simulink model "MS_test"  (R2024b)
settings: Solver=VariableStepAuto  StartTime=0.0  StopTime=10.0  RelTol=1e-3
undefined symbols (not defined in the file): dt, x0
settings Model: Creator=kasek  LastModifiedBy=kseki
settings RTWCC: GPUComputeCapability=3.5

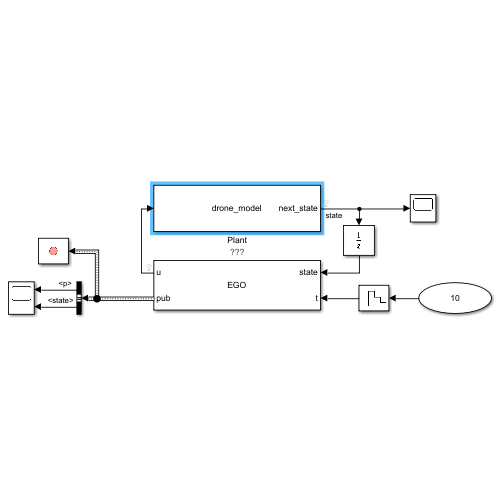
[thumbnail: Simulink's stored preview of the top-level diagram]
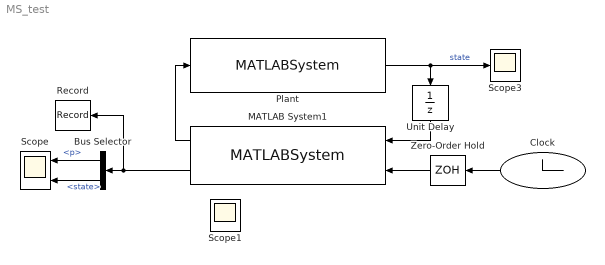
== system MS_test ==
  Bus Selector : BusSelector  OutputSignals=rresult.state.p,eresult.state
  Clock : Clock
  MATLAB System1 : MATLABSystem  System=EGO  SimulateUsing=Code generation
      mask Type: EGO
      mask Display:
      | disp('EGO');
      | port_label('input',1,'state');
      | port_label('input',2,'t');
      | port_label('output',1,'u');
      | port_label('output',2,'pub');
  Plant : MATLABSystem  System=drone_model  SimulateUsing=Code generation
      settings: AttributesFormatString=%<A>
      mask Type: drone_model
      mask Display:
      | disp('drone_model');
      | port_label('output',1,'next_state');
  Record : Record  FileSettingsInternal="{\"entries\":[{\"content\":{\"excelSettings\":{\"content\":{},\"type\":\"Streamout.ExcelSettings\"}},\"type\":\"Streamout.FileSettingStorage\",\"uuid\":\"\"}],\"packageUris\":[\"http:\\/\\/schema.mathworks.com\\/mf0\\/streamout_blocks\\/R2020a\"],\"version\":\"1.0\"}"  SignalsInternal="{\"entries\":[{\"content\":{\"signals\":[{\"content\":{\"blockPath\":[],\"dimensions\":[1,1],\"domain\":\"\",\"hasChildren\":true,\"lineColor\":\"#b746ff\",\"lineWidth\":2,\"port\":1,\"sid\":[\"\"],\"signalID\":1,\"signalName\":\"MATLAB System1:2\"},\"type\":\"RecordBlkView.Signal\",\"uuid\":\"\"},{\"content\":{\"blockPath\":[],\"dimensions\":[1],\"domain\":\"\",\"hasChildren\":true,\"lineColor\":\"#64d413\",\"lineWidth\":2,\"parentID\":1,\"port\":1,\"sid\":[\"\"],\"signalID\":2,\"signalName\":\"rresult\"},\"type\":\"RecordBlkView.Signal\",\"uuid\":\"\"},{\"content\":{\"blockPath\":[],\"dimensions\":[1],\"domain\":\"\",\"hasChildren\":true,\"lineColor\":\"#ff13a6\",\"lineWidth\":2,\"parentID\":2,\"port\":1,\"sid\":[\"\"],\"signalID\":3,\"signalName\":\"state\"},\"type\":\"RecordBlkView.Signal\",\"uuid\":\"\"},{\"content\":{\"blockPath\":[],\"dimensions\":[20,1],\"domain\":\"\",\"hasChildren\":true,\"lineColor\":\"#fe330a\",\"lineWidth\":2,\"parentID\":3,\"port\":1,\"sid\":[\"\"],\"signalID\":4,\"signalName\":\"MATLAB System1:2.rresult.state.xd\"},\"type\":\"RecordBlkView.Signal\",\"uuid\":\"\"},{\"content\":{\"blockPath\":[],\"channel\":[1,1],\"dimensions\":[20,1],\"domain\":\"\",\"leafPath\":\"MATLAB System1:2.rresult.state.xd\",\"lineColor\":\"#77ac30\",\"parentID\":4,\"plots\":[ 1 ],\"port\":1,\"sid\":[\"\"],\"signalID\":5,\"signalName\":\"MATLAB System1:2.rresult.state.xd\"},\"type\":\"RecordBlkView.Signal\",\"uuid\":\"\"},{\"content\":{\"blockPath\":[],\"dimensions\":[3,1],\"domain\":\"\",\"hasChildren\":true,\"lineColor\":\"#0072bd\",\"lineWidth\":2,\"parentID\":3,\"port\":1,\"sid\":[\"\"],\"signalID\":6,\"signalName\":\"MATLAB System1:2.rresult.state.p\"},\"type\":\"RecordBlkView.Signal\",\"uuid\":\"\"},{\"content\":{\"blockPath\":[],\"channel\":[1,1],\"dimensions\":[3,1],\"domain\":\"\",\"leafPath\":\"MATLAB System1:2.rresult.state.p\",\"lineColor\":\"#a2142f\",\"parentID\":6,\"plots\":[ 1 ],\"port\":1,\"sid\":[\"\"],\"signalID\":7,\"signalName\":\"MATLAB System1:2.rresult.state.p\"},\"type\":\"RecordBlkView.Signal\",\"uuid\":\"\"},{\"content\":{\"blockPath\":[],\"dimensions\":[3,1],\"domain\":\"\",\"hasChildren\":true,\"lineColor\":\"#edb120\",\"lineWidth\":2,\"parentID\":3,\"port\":1,\"sid\":[\"\"],\"signalID\":8,\"signalName\":\"MATLAB System1:2.rresult.state.v\"},\"type\":\"RecordBlkView.Signal\",\"uuid\":\"\"},{\"content\":{\"blockPath\":[],\"channel\":[1,1],\"dimensions\":[3,1],\"domain\":\"\",\"leafPath\":\"MATLAB System1:2.rresult.state.v\",\"lineColor\":\"#ff6929\",\"parentID\":8,\"plots\":[ 1 ],\"port\":1,\"sid\":[\"\"],\"signalID\":9,\"signalName\":\"MATLAB System1:2.rresult.state.v\"},\"type\":\"RecordBlkView.Signal\",\"uuid\":\"\"},{\"content\":{\"blockPath\":[],\"dimensions\":[3,1],\"domain\":\"\",\"hasChildren\":true,\"lineColor\":\"#77ac30\",\"lineWidth\":2,\"parentID\":3,\"port\":1,\"sid\":[\"\"],\"signalID\":10,\"signalName\":\"MATLAB System1:2.rresult.state.q\"},\"type\":\"RecordBlkView.Signal\",\"uuid\":\"\"},{\"content\":{\"blockPath\":[],\"channel\":[1,1],\"dimensions\":[3,1],\"domain\":\"\",\"leafPath\":\"MATLAB System1:2.rresult.state.q\",\"lineColor\":\"#64d413\",\"parentID\":10,\"plots\":[ 1 ],\"port\":1,\"sid\":[\"\"],\"signalID\":11,\"signalName\":\"MATLAB System1:2.rresult.state.q\"},\"type\":\"RecordBlkView.Signal\",\"uuid\":\"\"},{\"content\":{\"blockPath\":[],\"dimensions\":[1],\"domain\":\"\",\"hasChildren\":true,\"lineColor\":\"#a2142f\",\"lineWidth\":2,\"parentID\":1,\"port\":1,\"sid\":[\"\"],\"signalID\":12,\"signalName\":\"eresult\"},\"type\":\"RecordBlkView.Signal\",\"uuid\":\"\"},{\"content\":{\"blockPath\":[],\"dimensions\":[12,1],\"domain\":\"\",\"hasChildren\":true,\"lineColor\":\"#139fff\",\"lineWidth\":2,\"parentID\":12,\"port\":1,\"sid\":[\"\"],\"signalID\":13,\"signalName\":\"MATLAB System1:2.eresult.state\"},\"type\":\"RecordBlkView.Signal\",\"uuid\":\"\"},{\"content\":{\"blockPath\":[],\"channel\":[1,1],\"dimensions\":[12,1],\"domain\":\"\",\"leafPath\":\"MATLAB System1:2.eresult.state\",\"lineColor\":\"#22b573\",\"parentID\":13,\"plots\":[ 1 ],\"port\":1,\"sid\":[\"\"],\"signalID\":14,\"signalName\":\"MATLAB System1:2.eresult.state\"},\"type\":\"RecordBlkView.Signal\",\"uuid\":\"\"},{\"content\":{\"blockPath\":[],\"dimensions\":[12,12],\"domain\":\"\",\"hasChildren\":true,\"lineColor\":\"#b746ff\",\"lineWidth\":2,\"parentID\":12,\"port\":1,\"sid\":[\"\"],\"signalID\":15,\"signalName\":\"MATLAB System1:2.eresult.P\"},\"type\":\"RecordBlkView.Signal\",\"uuid\":\"\"},{\"content\":{\"blockPath\":[],\"channel\":[1,1],\"dimensions\":[12,12],\"domain\":\"\",\"leafPath\":\"MATLAB System1:2.eresult.P\",\"lineColor\":\"#d95319\",\"parentID\":15,\"plots\":[ 1 ],\"port\":1,\"sid\":[\"\"],\"signalID\":16,\"signalName\":\"MATLAB System1:2.eresult.P\"},\"type\":\"RecordBlkView.Signal\",\"uuid\":\"\"},{\"content\":{\"blockPath\":[],\"dimensions\":[1],\"domain\":\"\",\"hasChildren\":true,\"lineColor\":\"#ff13a6\",\"lineWidth\":2,\"parentID\":1,\"port\":1,\"sid\":[\"\"],\"signalID\":17,\"signalName\":\"cresult\"},\"type\":\"RecordBlkView.Signal\",\"uuid\":\"\"},{\"content\":{\"blockPath\":[],\"dimensions\":[4,1],\"domain\":\"\",\"hasChildren\":true,\"lineColor\":\"#fe330a\",\"lineWidth\":2,\"parentID\":17,\"port\":1,\"sid\":[\"\"],\"signalID\":18,\"signalName\":\"MATLAB System1:2.cresult.input\"},\"type\":\"RecordBlkView.Signal\",\"uuid\":\"\"},{\"content\":{\"blockPath\":[],\"channel\":[1,1],\"dimensions\":[4,1],\"domain\":\"\",\"leafPath\":\"MATLAB System1:2.cresult.input\",\"lineColor\":\"#77ac30\",\"parentID\":18,\"plots\":[ 1 ],\"port\":1,\"sid\":[\"\"],\"signalID\":19,\"signalName\":\"MATLAB System1:2.cresult.input\"},\"type\":\"RecordBlkView.Signal\",\"uuid\":\"\"},{\"content\":{\"blockPath\":[],\"channel\":[2,1],\"dimensions\":[3,1],\"domain\":\"\",\"leafPath\":\"MATLAB System1:2.rresult.state.p\",\"lineColor\":\"#ff6929\",\"parentID\":6,\"plots\":[ 1 ],\"port\":1,\"sid\":[\"\"],\"signalID\":20,\"signalName\":\"MATLAB System1:2.rresult.state.p\"},\"type\":\"RecordBlkView.Signal\",\"uuid\":\"\"},{\"content\":{\"blockPath\":[],\"channel\":[3,1],\"dimensions\":[3,1],\"domain\":\"\",\"leafPath\":\"MATLAB System1:2.rresult.state.p\",\"lineColor\":\"#b746ff\",\"parentID\":6,\"plots\":[ 1 ],\"port\":1,\"sid\":[\"\"],\"signalID\":21,\"signalName\":\"MATLAB System1:2.rresult.state.p\"},\"type\":\"RecordBlkView.Signal\",\"uuid\":\"\"},{\"content\":{\"blockPath\":[],\"channel\":[2,1],\"dimensions\":[3,1],\"domain\":\"\",\"leafPath\":\"MATLAB System1:2.rresult.state.v\",\"lineColor\":\"#64d413\",\"parentID\":8,\"plots\":[ 1 ],\"port\":1,\"sid\":[\"\"],\"signalID\":22,\"signalName\":\"MATLAB System1:2.rresult.state.v\"},\"type\":\"RecordBlkView.Signal\",\"uuid\":\"\"},{\"content\":{\"blockPath\":[],\"channel\":[3,1],\"dimensions\":[3,1],\"domain\":\"\",\"leafPath\":\"MATLAB System1:2.rresult.state.v\",\"lineColor\":\"#ff13a6\",\"parentID\":8,\"plots\":[ 1 ],\"port\":1,\"sid\":[\"\"],\"signalID\":23,\"signalName\":\"MATLAB System1:2.rresult.state.v\"},\"type\":\"RecordBlkView.Signal\",\"uuid\":\"\"},{\"content\":{\"blockPath\":[],\"channel\":[2,1],\"dimensions\":[3,1],\"domain\":\"\",\"leafPath\":\"MATLAB System1:2.rresult.state.q\",\"lineColor\":\"#fe330a\",\"parentID\":10,\"plots\":[ 1 ],\"port\":1,\"sid\":[\"\"],\"signalID\":24,\"signalName\":\"MATLAB System1:2.rresult.state.q\"},\"type\":\"RecordBlkView.Signal\",\"uuid\":\"\"},{\"content\":{\"blockPath\":[],\"channel\":[3,1],\"dimensions\":[3,1],\"domain\":\"\",\"leafPath\":\"MATLAB System1:2.rresult.state.q\",\"lineColor\":\"#22b573\",\"parentID\":10,\"plots\":[ 1 ],\"port\":1,\"sid\":[\"\"],\"signalID\":25,\"signalName\":\"MATLAB System1:2.rresult.state.q\"},\"type\":\"RecordBlkView.Signal\",\"uuid\":\"\"},{\"content\":{\"blockPath\":[],\"channel\":[2,1],\"dimensions\":[4,1],\"domain\":\"\",\"leafPath\":\"MATLAB System1:2.cresult.input\",\"lineColor\":\"#0072bd\",\"parentID\":18,\"plots\":[ 1 ],\"port\":1,\"sid\":[\"\"],\"signalID\":26,\"signalName\":\"MATLAB System1:2.cresult.input\"},\"type\":\"RecordBlkView.Signal\",\"uuid\":\"\"},{\"content\":{\"blockPath\":[],\"channel\":[3,1],\"dimensions\":[4,1],\"domain\":\"\",\"leafPath\":\"MATLAB System1:2.cresult.input\",\"lineColor\":\"#d95319\",\"parentID\":18,\"plots\":[ 1 ],\"port\":1,\"sid\":[\"\"],\"signalID\":27,\"signalName\":\"MATLAB System1:2.cresult.input\"},\"type\":\"RecordBlkView.Signal\",\"uuid\":\"\"},{\"content\":{\"blockPath\":[],\"channel\":[4,1],\"dimensions\":[4,1],\"domain\":\"\",\"leafPath\":\"MATLAB System1:2.cresult.input\",\"lineColor\":\"#edb120\",\"parentID\":18,\"plots\":[ 1 ],\"port\":1,\"sid\":[\"\"],\"signalID\":28,\"signalName\":\"MATLAB System1:2.cresult.input\"},\"type\":\"RecordBlkView.Signal\",\"uuid\":\"\"},{\"content\":{\"blockPath\":[],\"channel\":[2,1],\"dimensions\":[20,1],\"domain\":\"\",\"leafPath\":\"MATLAB System1:2.rresult.state.xd\",\"lineColor\":\"#fe330a\",\"lineWidth\":2,\"parentID\":4,\"plots\":[ 1 ],\"port\":1,\"sid\":[\"\"],\"signalID\":29,\"signalName\":\"MATLAB System1:2.rresult.state.xd\"},\"type\":\"RecordBlkView.Signal\",\"uuid\":\"\"},{\"content\":{\"blockPath\":[],\"channel\":[3,1],\"dimensions\":[20,1],\"domain\":\"\",\"leafPath\":\"MATLAB System1:2.rresult.state.xd\",\"lineColor\":\"#22b573\",\"lineWidth\":2,\"parentID\":4,\"plots\":[ 1 ],\"port\":1,\"sid\":[\"\"],\"signalID\":30,\"signalName\":\"MATLAB System1:2.rresult.state.xd\"},\"type\":\"RecordBlkView.Signal\",\"uuid\":\"\"},{\"content\":{\"blockPath\":[],\"channel\":[4,1],\"dimensions\":[20,1],\"domain\":\"\",\"leafPath\":\"MATLAB System1:2.rresult.state.xd\",\"lineColor\":\"#0072bd\",\"lineWidth\":2,\"parentID\":4,\"plots\":[ 1 ],\"port\":1,\"sid\":[\"\"],\"signalID\":31,\"signalName\":\"MATLAB System1:2.rresult.state.xd\"},\"type\":\"RecordBlkView.Signal\",\"uuid\":\"\"},{\"content\":{\"blockPath\":[],\"channel\":[5,1],\"dimensions\":[20,1],\"domain\":\"\",\"leafPath\":\"MATLAB System1:2.rresult.state.xd\",\"lineColor\":\"#d95319\",\"lineWidth\":2,\"parentID\":4,\"port\":1,\"sid\":[\"\"],\"signalID\":32,\"signalName\":\"MATLAB System1:2.rresult.state.xd\"},\"type\":\"RecordBlkView.Signal\",\"uuid\":\"\"},{\"content\":{\"blockPath\":[],\"channel\":[6,1],\"dimensions\":[20,1],\"domain\":\"\",\"leafPath\":\"MATLAB System1:2.rresult.state.xd\",\"lineColor\":\"#edb120\",\"lineWidth\":2,\"parentID\":4,\"port\":1,\"sid\":[\"\"],\"signalID\":33,\"signalName\":\"MATLAB System1:2.rresult.state.xd\"},\"type\":\"RecordBlkView.Signal\",\"uuid\":\"\"},{\"content\":{\"blockPath\":[],\"channel\":[7,1],\"dimensions\":[20,1],\"domain\":\"\",\"leafPath\":\"MATLAB System1:2.rresult.state.xd\",\"lineColor\":\"#7e2f8e\",\"lineWidth\":2,\"parentID\":4,\"port\":1,\"sid\":[\"\"],\"signalID\":34,\"signalName\":\"MATLAB System1:2.rresult.state.xd\"},\"type\":\"RecordBlkView.Signal\",\"uuid\":\"\"},{\"content\":{\"blockPath\":[],\"channel\":[8,1],\"dimensions\":[20,1],\"domain\":\"\",\"leafPath\":\"MATLAB System1:2.rresult.state.xd\",\"lineColor\":\"#77ac30\",\"lineWidth\":2,\"parentID\":4,\"port\":1,\"sid\":[\"\"],\"signalID\":35,\"signalName\":\"MATLAB System1:2.rresult.state.xd\"},\"type\":\"RecordBlkView.Signal\",\"uuid\":\"\"},{\"content\":{\"blockPath\":[],\"channel\":[9,1],\"dimensions\":[20,1],\"domain\":\"\",\"leafPath\":\"MATLAB System1:2.rresult.state.xd\",\"lineColor\":\"#4dbeee\",\"lineWidth\":2,\"parentID\":4,\"port\":1,\"sid\":[\"\"],\"signalID\":36,\"signalName\":\"MATLAB System1:2.rresult.state.xd\"},\"type\":\"RecordBlkView.Signal\",\"uuid\":\"\"},{\"content\":{\"blockPath\":[],\"channel\":[10,1],\"dimensions\":[20,1],\"domain\":\"\",\"leafPath\":\"MATLAB System1:2.rresult.state.xd\",\"lineColor\":\"#a2142f\",\"lineWidth\":2,\"parentID\":4,\"port\":1,\"sid\":[\"\"],\"signalID\":37,\"signalName\":\"MATLAB System1:2.rresult.state.xd\"},\"type\":\"RecordBlkView.Signal\",\"uuid\":\"\"},{\"content\":{\"blockPath\":[],\"channel\":[11,1],\"dimensions\":[20,1],\"domain\":\"\",\"leafPath\":\"MATLAB System1:2.rresult.state.xd\",\"lineColor\":\"#139fff\",\"lineWidth\":2,\"parentID\":4,\"port\":1,\"sid\":[\"\"],\"signalID\":38,\"signalName\":\"MATLAB System1:2.rresult.state.xd\"},\"type\":\"RecordBlkView.Signal\",\"uuid\":\"\"},{\"content\":{\"blockPath\":[],\"channel\":[12,1],\"dimensions\":[20,1],\"domain\":\"\",\"leafPath\":\"MATLAB System1:2.rresult.state.xd\",\"lineColor\":\"#ff6929\",\"lineWidth\":2,\"parentID\":4,\"port\":1,\"sid\":[\"\"],\"signalID\":39,\"signalName\":\"MATLAB System1:2.rresult.state.xd\"},\"type\":\"RecordBlkView.Signal\",\"uuid\":\"\"},{\"content\":{\"blockPath\":[],\"channel\":[13,1],\"dimensions\":[20,1],\"domain\":\"\",\"leafPath\":\"MATLAB System1:2.rresult.state.xd\",\"lineColor\":\"#b746ff\",\"lineWidth\":2,\"parentID\":4,\"port\":1,\"sid\":[\"\"],\"signalID\":40,\"signalName\":\"MATLAB System1:2.rresult.state.xd\"},\"type\":\"RecordBlkView.Signal\",\"uuid\":\"\"},{\"content\":{\"blockPath\":[],\"channel\":[14,1],\"dimensions\":[20,1],\"domain\":\"\",\"leafPath\":\"MATLAB System1:2.rresult.state.xd\",\"lineColor\":\"#64d413\",\"lineWidth\":2,\"parentID\":4,\"port\":1,\"sid\":[\"\"],\"signalID\":41,\"signalName\":\"MATLAB System1:2.rresult.state.xd\"},\"type\":\"RecordBlkView.Signal\",\"uuid\":\"\"},{\"content\":{\"blockPath\":[],\"channel\":[15,1],\"dimensions\":[20,1],\"domain\":\"\",\"leafPath\":\"MATLAB System1:2.rresult.state.xd\",\"lineColor\":\"#ff13a6\",\"lineWidth\":2,\"parentID\":4,\"port\":1,\"sid\":[\"\"],\"signalID\":42,\"signalName\":\"MATLAB System1:2.rresult.state.xd\"},\"type\":\"RecordBlkView.Signal\",\"uuid\":\"\"},{\"content\":{\"blockPath\":[],\"channel\":[16,1],\"dimensions\":[20,1],\"domain\":\"\",\"leafPath\":\"MATLAB System1:2.rresult.state.xd\",\"lineColor\":\"#fe330a\",\"lineWidth\":2,\"parentID\":4,\"port\":1,\"sid\":[\"\"],\"signalID\":43,\"signalName\":\"MATLAB System1:2.rresult.state.xd\"},\"type\":\"RecordBlkView.Signal\",\"uuid\":\"\"},{\"content\":{\"blockPath\":[],\"channel\":[17,1],\"dimensions\":[20,1],\"domain\":\"\",\"leafPath\":\"MATLAB System1:2.rresult.state.xd\",\"lineColor\":\"#22b573\",\"lineWidth\":2,\"parentID\":4,\"port\":1,\"sid\":[\"\"],\"signalID\":44,\"signalName\":\"MATLAB System1:2.rresult.state.xd\"},\"type\":\"RecordBlkView.Signal\",\"uuid\":\"\"},{\"content\":{\"blockPath\":[],\"channel\":[18,1],\"dimensions\":[20,1],\"domain\":\"\",\"leafPath\":\"MATLAB System1:2.rresult.state.xd\",\"lineColor\":\"#0072bd\",\"lineWidth\":2,\"parentID\":4,\"port\":1,\"sid\":[\"\"],\"signalID\":45,\"signalName\":\"MATLAB System1:2.rresult.state.xd\"},\"type\":\"RecordBlkView.Signal\",\"uuid\":\"\"},{\"content\":{\"blockPath\":[],\"channel\":[19,1],\"dimensions\":[20,1],\"domain\":\"\",\"leafPath\":\"MATLAB System1:2.rresult.state.xd\",\"lineColor\":\"#d95319\",\"lineWidth\":2,\"parentID\":4,\"port\":1,\"sid\":[\"\"],\"signalID\":46,\"signalName\":\"MATLAB System1:2.rresult.state.xd\"},\"type\":\"RecordBlkView.Signal\",\"uuid\":\"\"},{\"content\":{\"blockPath\":[],\"channel\":[20,1],\"dimensions\":[20,1],\"domain\":\"\",\"leafPath\":\"MATLAB System1:2.rresult.state.xd\",\"lineColor\":\"#edb120\",\"lineWidth\":2,\"parentID\":4,\"port\":1,\"sid\":[\"\"],\"signalID\":47,\"signalName\":\"MATLAB System1:2.rresult.state.xd\"},\"type\":\"RecordBlkView.Signal\",\"uuid\":\"\"},{\"content\":{\"blockPath\":[],\"channel\":[2,1],\"dimensions\":[12,1],\"domain\":\"\",\"leafPath\":\"MATLAB System1:2.eresult.state\",\"lineColor\":\"#7e2f8e\",\"lineWidth\":2,\"parentID\":13,\"plots\":[ 1 ],\"port\":1,\"sid\":[\"\"],\"signalID\":48,\"signalName\":\"MATLAB System1:2.eresult.state\"},\"type\":\"RecordBlkView.Signal\",\"uuid\":\"\"},{\"content\":{\"blockPath\":[],\"channel\":[3,1],\"dimensions\":[12,1],\"domain\":\"\",\"leafPath\":\"MATLAB System1:2.eresult.state\",\"lineColor\":\"#77ac30\",\"lineWidth\":2,\"parentID\":13,\"plots\":[ 1 ],\"port\":1,\"sid\":[\"\"],\"signalID\":49,\"signalName\":\"MATLAB System1:2.eresult.state\"},\"type\":\"RecordBlkView.Signal\",\"uuid\":\"\"},{\"content\":{\"blockPath\":[],\"channel\":[4,1],\"dimensions\":[12,1],\"domain\":\"\",\"leafPath\":\"MATLAB System1:2.eresult.state\",\"lineColor\":\"#4dbeee\",\"lineWidth\":2,\"parentID\":13,\"plots\":[ 1 ],\"port\":1,\"sid\":[\"\"],\"signalID\":50,\"signalName\":\"MATLAB System1:2.eresult.state\"},\"type\":\"RecordBlkView.Signal\",\"uuid\":\"\"},{\"content\":{\"blockPath\":[],\"channel\":[5,1],\"dimensions\":[12,1],\"domain\":\"\",\"leafPath\":\"MATLAB System1:2.eresult.state\",\"lineColor\":\"#a2142f\",\"lineWidth\":2,\"parentID\":13,\"port\":1,\"sid\":[\"\"],\"signalID\":51,\"signalName\":\"MATLAB System1:2.eresult.state\"},\"type\":\"RecordBlkView.Signal\",\"uuid\":\"\"},{\"content\":{\"blockPath\":[],\"channel\":[6,1],\"dimensions\":[12,1],\"domain\":\"\",\"leafPath\":\"MATLAB System1:2.eresult.state\",\"lineColor\":\"#139fff\",\"lineWidth\":2,\"parentID\":13,\"port\":1,\"sid\":[\"\"],\"signalID\":52,\"signalName\":\"MATLAB System1:2.eresult.state\"},\"type\":\"RecordBlkView.Signal\",\"uuid\":\"\"},{\"content\":{\"blockPath\":[],\"channel\":[7,1],\"dimensions\":[12,1],\"domain\":\"\",\"leafPath\":\"MATLAB System1:2.eresult.state\",\"lineColor\":\"#ff6929\",\"lineWidth\":2,\"parentID\":13,\"port\":1,\"sid\":[\"\"],\"signalID\":53,\"signalName\":\"MATLAB System1:2.eresult.state\"},\"type\":\"RecordBlkView.Signal\",\"uuid\":\"\"},{\"content\":{\"blockPath\":[],\"channel\":[8,1],\"dimensions\":[12,1],\"domain\":\"\",\"leafPath\":\"MATLAB System1:2.eresult.state\",\"lineColor\":\"#b746ff\",\"lineWidth\":2,\"parentID\":13,\"port\":1,\"sid\":[\"\"],\"signalID\":54,\"signalName\":\"MATLAB System1:2.eresult.state\"},\"type\":\"RecordBlkView.Signal\",\"uuid\":\"\"},{\"content\":{\"blockPath\":[],\"channel\":[9,1],\"dimensions\":[12,1],\"domain\":\"\",\"leafPath\":\"MATLAB System1:2.eresult.state\",\"lineColor\":\"#64d413\",\"lineWidth\":2,\"parentID\":13,\"port\":1,\"sid\":[\"\"],\"signalID\":55,\"signalName\":\"MATLAB System1:2.eresult.state\"},\"type\":\"RecordBlkView.Signal\",\"uuid\":\"\"},{\"content\":{\"blockPath\":[],\"channel\":[10,1],\"dimensions\":[12,1],\"domain\":\"\",\"leafPath\":\"MATLAB System1:2.eresult.state\",\"lineColor\":\"#ff13a6\",\"lineWidth\":2,\"parentID\":13,\"port\":1,\"sid\":[\"\"],\"signalID\":56,\"signalName\":\"MATLAB System1:2.eresult.state\"},\"type\":\"RecordBlkView.Signal\",\"uuid\":\"\"},{\"content\":{\"blockPath\":[],\"channel\":[11,1],\"dimensions\":[12,1],\"domain\":\"\",\"leafPath\":\"MATLAB System1:2.eresult.state\",\"lineColor\":\"#fe330a\",\"lineWidth\":2,\"parentID\":13,\"port\":1,\"sid\":[\"\"],\"signalID\":57,\"signalName\":\"MATLAB System1:2.eresult.state\"},\"type\":\"RecordBlkView.Signal\",\"uuid\":\"\"},{\"content\":{\"blockPath\":[],\"channel\":[12,1],\"dimensions\":[12,1],\"domain\":\"\",\"leafPath\":\"MATLAB System1:2.eresult.state\",\"lineColor\":\"#22b573\",\"lineWidth\":2,\"parentID\":13,\"port\":1,\"sid\":[\"\"],\"signalID\":58,\"signalName\":\"MATLAB System1:2.eresult.state\"},\"type\":\"RecordBlkView.Signal\",\"uuid\":\"\"},{\"content\":{\"blockPath\":[],\"channel\":[2,1],\"dimensions\":[12,12],\"domain\":\"\",\"leafPath\":\"MATLAB System1:2.eresult.P\",\"lineColor\":\"#0072bd\",\"lineWidth\":2,\"parentID\":15,\"plots\":[ 1 ],\"port\":1,\"sid\":[\"\"],\"signalID\":59,\"signalName\":\"MATLAB System1:2.eresult.P\"},\"type\":\"RecordBlkView.Signal\",\"uuid\":\"\"},{\"content\":{\"blockPath\":[],\"channel\":[3,1],\"dimensions\":[12,12],\"domain\":\"\",\"leafPath\":\"MATLAB System1:2.eresult.P\",\"lineColor\":\"#d95319\",\"lineWidth\":2,\"parentID\":15,\"plots\":[ 1 ],\"port\":1,\"sid\":[\"\"],\"signalID\":60,\"signalName\":\"MATLAB System1:2.eresult.P\"},\"type\":\"RecordBlkView.Signal\",\"uuid\":\"\"},{\"content\":{\"blockPath\":[],\"channel\":[4,1],\"dimensions\":[12,12],\"domain\":\"\",\"leafPath\":\"MATLAB System1:2.eresult.P\",\"lineColor\":\"#edb120\",\"lineWidth\":2,\"parentID\":15,\"plots\":[ 1 ],\"port\":1,\"sid\":[\"\"],\"signalID\":61,\"signalName\":\"MATLAB System1:2.eresult.P\"},\"type\":\"RecordBlkView.Signal\",\"uuid\":\"\"},{\"content\":{\"blockPath\":[],\"channel\":[5,1],\"dimensions\":[12,12],\"domain\":\"\",\"leafPath\":\"MATLAB System1:2.eresult.P\",\"lineColor\":\"#7e2f8e\",\"lineWidth\":2,\"parentID\":15,\"port\":1,\"sid\":[\"\"],\"signalID\":62,\"signalName\":\"MATLAB System1:2.eresult.P\"},\"type\":\"RecordBlkView.Signal\",\"uuid\":\"\"},{\"content\":{\"blockPath\":[],\"channel\":[6,1],\"dimensions\":[12,12],\"domain\":\"\",\"leafPath\":\"MATLAB System1:2.eresult.P\",\"lineColor\":\"#77ac30\",\"lineWidth\":2,\"parentID\":15,\"port\":1,\"sid\":[\"\"],\"signalID\":63,\"signalName\":\"MATLAB System1:2.eresult.P\"},\"type\":\"RecordBlkView.Signal\",\"uuid\":\"\"},{\"content\":{\"blockPath\":[],\"channel\":[7,1],\"dimensions\":[12,12],\"domain\":\"\",\"leafPath\":\"MATLAB System1:2.eresult.P\",\"lineColor\":\"#4dbeee\",\"lineWidth\":2,\"parentID\":15,\"port\":1,\"sid\":[\"\"],\"signalID\":64,\"signalName\":\"MATLAB System1:2.eresult.P\"},\"type\":\"RecordBlkView.Signal\",\"uuid\":\"\"},{\"content\":{\"blockPath\":[],\"channel\":[8,1],\"dimensions\":[12,12],\"domain\":\"\",\"leafPath\":\"MATLAB System1:2.eresult.P\",\"lineColor\":\"#a2142f\",\"lineWidth\":2,\"parentID\":15,\"port\":1,\"sid\":[\"\"],\"signalID\":65,\"signalName\":\"MATLAB System1:2.eresult.P\"},\"type\":\"RecordBlkView.Signal\",\"uuid\":\"\"},{\"content\":{\"blockPath\":[],\"channel\":[9,1],\"dimensions\":[12,12],\"domain\":\"\",\"leafPath\":\"MATLAB System1:2.eresult.P\",\"lineColor\":\"#139fff\",\"lineWidth\":2,\"parentID\":15,\"port\":1,\"sid\":[\"\"],\"signalID\":66,\"signalName\":\"MATLAB System1:2.eresult.P\"},\"type\":\"RecordBlkView.Signal\",\"uuid\":\"\"},{\"content\":{\"blockPath\":[],\"channel\":[10,1],\"dimensions\":[12,12],\"domain\":\"\",\"leafPath\":\"MATLAB System1:2.eresult.P\",\"lineColor\":\"#ff6929\",\"lineWidth\":2,\"parentID\":15,\"port\":1,\"sid\":[\"\"],\"signalID\":67,\"signalName\":\"MATLAB System1:2.eresult.P\"},\"type\":\"RecordBlkView.Signal\",\"uuid\":\"\"},{\"content\":{\"blockPath\":[],\"channel\":[11,1],\"dimensions\":[12,12],\"domain\":\"\",\"leafPath\":\"MATLAB System1:2.eresult.P\",\"lineColor\":\"#b746ff\",\"lineWidth\":2,\"parentID\":15,\"port\":1,\"sid\":[\"\"],\"signalID\":68,\"signalName\":\"MATLAB System1:2.eresult.P\"},\"type\":\"RecordBlkView.Signal\",\"uuid\":\"\"},{\"content\":{\"blockPath\":[],\"channel\":[12,1],\"dimensions\":[12,12],\"domain\":\"\",\"leafPath\":\"MATLAB System1:2.eresult.P\",\"lineColor\":\"#64d413\",\"lineWidth\":2,\"parentID\":15,\"port\":1,\"sid\":[\"\"],\"signalID\":69,\"signalName\":\"MATLAB System1:2.eresult.P\"},\"type\":\"RecordBlkView.Signal\",\"uuid\":\"\"},{\"content\":{\"blockPath\":[],\"channel\":[1,2],\"dimensions\":[12,12],\"domain\":\"\",\"leafPath\":\"MATLAB System1:2.eresult.P\",\"lineColor\":\"#ff13a6\",\"lineWidth\":2,\"parentID\":15,\"port\":1,\"sid\":[\"\"],\"signalID\":70,\"signalName\":\"MATLAB System1:2.eresult.P\"},\"type\":\"RecordBlkView.Signal\",\"uuid\":\"\"},{\"content\":{\"blockPath\":[],\"channel\":[2,2],\"dimensions\":[12,12],\"domain\":\"\",\"leafPath\":\"MATLAB System1:2.eresult.P\",\"lineColor\":\"#fe330a\",\"lineWidth\":2,\"parentID\":15,\"port\":1,\"sid\":[\"\"],\"signalID\":71,\"signalName\":\"MATLAB System1:2.eresult.P\"},\"type\":\"RecordBlkView.Signal\",\"uuid\":\"\"},{\"content\":{\"blockPath\":[],\"channel\":[3,2],\"dimensions\":[12,12],\"domain\":\"\",\"leafPath\":\"MATLAB System1:2.eresult.P\",\"lineColor\":\"#22b573\",\"lineWidth\":2,\"parentID\":15,\"port\":1,\"sid\":[\"\"],\"signalID\":72,\"signalName\":\"MATLAB System1:2.eresult.P\"},\"type\":\"RecordBlkView.Signal\",\"uuid\":\"\"},{\"content\":{\"blockPath\":[],\"channel\":[4,2],\"dimensions\":[12,12],\"domain\":\"\",\"leafPath\":\"MATLAB System1:2.eresult.P\",\"lineColor\":\"#0072bd\",\"lineWidth\":2,\"parentID\":15,\"port\":1,\"sid\":[\"\"],\"signalID\":73,\"signalName\":\"MATLAB System1:2.eresult.P\"},\"type\":\"RecordBlkView.Signal\",\"uuid\":\"\"},{\"content\":{\"blockPath\":[],\"channel\":[5,2],\"dimensions\":[12,12],\"domain\":\"\",\"leafPath\":\"MATLAB System1:2.eresult.P\",\"lineColor\":\"#d95319\",\"lineWidth\":2,\"parentID\":15,\"port\":1,\"sid\":[\"\"],\"signalID\":74,\"signalName\":\"MATLAB System1:2.eresult.P\"},\"type\":\"RecordBlkView.Signal\",\"uuid\":\"\"},{\"content\":{\"blockPath\":[],\"channel\":[6,2],\"dimensions\":[12,12],\"domain\":\"\",\"leafPath\":\"MATLAB System1:2.eresult.P\",\"lineColor\":\"#edb120\",\"lineWidth\":2,\"parentID\":15,\"port\":1,\"sid\":[\"\"],\"signalID\":75,\"signalName\":\"MATLAB System1:2.eresult.P\"},\"type\":\"RecordBlkView.Signal\",\"uuid\":\"\"},{\"content\":{\"blockPath\":[],\"channel\":[7,2],\"dimensions\":[12,12],\"domain\":\"\",\"leafPath\":\"MATLAB System1:2.eresult.P\",\"lineColor\":\"#7e2f8e\",\"lineWidth\":2,\"parentID\":15,\"port\":1,\"sid\":[\"\"],\"signalID\":76,\"signalName\":\"MATLAB System1:2.eresult.P\"},\"type\":\"RecordBlkView.Signal\",\"uuid\":\"\"},{\"content\":{\"blockPath\":[],\"channel\":[8,2],\"dimensions\":[12,12],\"domain\":\"\",\"leafPath\":\"MATLAB System1:2.eresult.P\",\"lineColor\":\"#77ac30\",\"lineWidth\":2,\"parentID\":15,\"port\":1,\"sid\":[\"\"],\"signalID\":77,\"signalName\":\"MATLAB System1:2.eresult.P\"},\"type\":\"RecordBlkView.Signal\",\"uuid\":\"\"},{\"content\":{\"blockPath\":[],\"channel\":[9,2],\"dimensions\":[12,12],\"domain\":\"\",\"leafPath\":\"MATLAB System1:2.eresult.P\",\"lineColor\":\"#4dbeee\",\"lineWidth\":2,\"parentID\":15,\"port\":1,\"sid\":[\"\"],\"signalID\":78,\"signalName\":\"MATLAB System1:2.eresult.P\"},\"type\":\"RecordBlkView.Signal\",\"uuid\":\"\"},{\"content\":{\"blockPath\":[],\"channel\":[10,2],\"dimensions\":[12,12],\"domain\":\"\",\"leafPath\":\"MATLAB System1:2.eresult.P\",\"lineColor\":\"#a2142f\",\"lineWidth\":2,\"parentID\":15,\"port\":1,\"sid\":[\"\"],\"signalID\":79,\"signalName\":\"MATLAB System1:2.eresult.P\"},\"type\":\"RecordBlkView.Signal\",\"uuid\":\"\"},{\"content\":{\"blockPath\":[],\"channel\":[11,2],\"dimensions\":[12,12],\"domain\":\"\",\"leafPath\":\"MATLAB System1:2.eresult.P\",\"lineColor\":\"#139fff\",\"lineWidth\":2,\"parentID\":15,\"port\":1,\"sid\":[\"\"],\"signalID\":80,\"signalName\":\"MATLAB System1:2.eresult.P\"},\"type\":\"RecordBlkView.Signal\",\"uuid\":\"\"},{\"content\":{\"blockPath\":[],\"channel\":[12,2],\"dimensions\":[12,12],\"domain\":\"\",\"leafPath\":\"MATLAB System1:2.eresult.P\",\"lineColor\":\"#ff6929\",\"lineWidth\":2,\"parentID\":15,\"port\":1,\"sid\":[\"\"],\"signalID\":81,\"signalName\":\"MATLAB System1:2.eresult.P\"},\"type\":\"RecordBlkView.Signal\",\"uuid\":\"\"},{\"content\":{\"blockPath\":[],\"channel\":[1,3],\"dimensions\":[12,12],\"domain\":\"\",\"leafPath\":\"MATLAB System1:2.eresult.P\",\"lineColor\":\"#b746ff\",\"lineWidth\":2,\"parentID\":15,\"port\":1,\"sid\":[\"\"],\"signalID\":82,\"signalName\":\"MATLAB System1:2.eresult.P\"},\"type\":\"RecordBlkView.Signal\",\"uuid\":\"\"},{\"content\":{\"blockPath\":[],\"channel\":[2,3],\"dimensions\":[12,12],\"domain\":\"\",\"leafPath\":\"MATLAB System1:2.eresult.P\",\"lineColor\":\"#64d413\",\"lineWidth\":2,\"parentID\":15,\"port\":1,\"sid\":[\"\"],\"signalID\":83,\"signalName\":\"MATLAB System1:2.eresult.P\"},\"type\":\"RecordBlkView.Signal\",\"uuid\":\"\"},{\"content\":{\"blockPath\":[],\"channel\":[3,3],\"dimensions\":[12,12],\"domain\":\"\",\"leafPath\":\"MATLAB System1:2.eresult.P\",\"lineColor\":\"#ff13a6\",\"lineWidth\":2,\"parentID\":15,\"port\":1,\"sid\":[\"\"],\"signalID\":84,\"signalName\":\"MATLAB System1:2.eresult.P\"},\"type\":\"RecordBlkView.Signal\",\"uuid\":\"\"},{\"content\":{\"blockPath\":[],\"channel\":[4,3],\"dimensions\":[12,12],\"domain\":\"\",\"leafPath\":\"MATLAB System1:2.eresult.P\",\"lineColor\":\"#fe330a\",\"lineWidth\":2,\"parentID\":15,\"port\":1,\"sid\":[\"\"],\"signalID\":85,\"signalName\":\"MATLAB System1:2.eresult.P\"},\"type\":\"RecordBlkView.Signal\",\"uuid\":\"\"},{\"content\":{\"blockPath\":[],\"channel\":[5,3],\"dimensions\":[12,12],\"domain\":\"\",\"leafPath\":\"MATLAB System1:2.eresult.P\",\"lineColor\":\"#22b573\",\"lineWidth\":2,\"parentID\":15,\"port\":1,\"sid\":[\"\"],\"signalID\":86,\"signalName\":\"MATLAB System1:2.eresult.P\"},\"type\":\"RecordBlkView.Signal\",\"uuid\":\"\"},{\"content\":{\"blockPath\":[],\"channel\":[6,3],\"dimensions\":[12,12],\"domain\":\"\",\"leafPath\":\"MATLAB System1:2.eresult.P\",\"lineColor\":\"#0072bd\",\"lineWidth\":2,\"parentID\":15,\"port\":1,\"sid\":[\"\"],\"signalID\":87,\"signalName\":\"MATLAB System1:2.eresult.P\"},\"type\":\"RecordBlkView.Signal\",\"uuid\":\"\"},{\"content\":{\"blockPath\":[],\"channel\":[7,3],\"dimensions\":[12,12],\"domain\":\"\",\"leafPath\":\"MATLAB System1:2.eresult.P\",\"lineColor\":\"#d95319\",\"lineWidth\":2,\"parentID\":15,\"port\":1,\"sid\":[\"\"],\"signalID\":88,\"signalName\":\"MATLAB System1:2.eresult.P\"},\"type\":\"RecordBlkView.Signal\",\"uuid\":\"\"},{\"content\":{\"blockPath\":[],\"channel\":[8,3],\"dimensions\":[12,12],\"domain\":\"\",\"leafPath\":\"MATLAB System1:2.eresult.P\",\"lineColor\":\"#edb120\",\"lineWidth\":2,\"parentID\":15,\"port\":1,\"sid\":[\"\"],\"signalID\":89,\"signalName\":\"MATLAB System1:2.eresult.P\"},\"type\":\"RecordBlkView.Signal\",\"uuid\":\"\"},{\"content\":{\"blockPath\":[],\"channel\":[9,3],\"dimensions\":[12,12],\"domain\":\"\",\"leafPath\":\"MATLAB System1:2.eresult.P\",\"lineColor\":\"#7e2f8e\",\"lineWidth\":2,\"parentID\":15,\"port\":1,\"sid\":[\"\"],\"signalID\":90,\"signalName\":\"MATLAB System1:2.eresult.P\"},\"type\":\"RecordBlkView.Signal\",\"uuid\":\"\"},{\"content\":{\"blockPath\":[],\"channel\":[10,3],\"dimensions\":[12,12],\"domain\":\"\",\"leafPath\":\"MATLAB System1:2.eresult.P\",\"lineColor\":\"#77ac30\",\"lineWidth\":2,\"parentID\":15,\"port\":1,\"sid\":[\"\"],\"signalID\":91,\"signalName\":\"MATLAB System1:2.eresult.P\"},\"type\":\"RecordBlkView.Signal\",\"uuid\":\"\"},{\"content\":{\"blockPath\":[],\"channel\":[11,3],\"dimensions\":[12,12],\"domain\":\"\",\"leafPath\":\"MATLAB System1:2.eresult.P\",\"lineColor\":\"#4dbeee\",\"lineWidth\":2,\"parentID\":15,\"port\":1,\"sid\":[\"\"],\"signalID\":92,\"signalName\":\"MATLAB System1:2.eresult.P\"},\"type\":\"RecordBlkView.Signal\",\"uuid\":\"\"},{\"content\":{\"blockPath\":[],\"channel\":[12,3],\"dimensions\":[12,12],\"domain\":\"\",\"leafPath\":\"MATLAB System1:2.eresult.P\",\"lineColor\":\"#a2142f\",\"lineWidth\":2,\"parentID\":15,\"port\":1,\"sid\":[\"\"],\"signalID\":93,\"signalName\":\"MATLAB System1:2.eresult.P\"},\"type\":\"RecordBlkView.Signal\",\"uuid\":\"\"},{\"content\":{\"blockPath\":[],\"channel\":[1,4],\"dimensions\":[12,12],\"domain\":\"\",\"leafPath\":\"MATLAB System1:2.eresult.P\",\"lineColor\":\"#139fff\",\"lineWidth\":2,\"parentID\":15,\"port\":1,\"sid\":[\"\"],\"signalID\":94,\"signalName\":\"MATLAB System1:2.eresult.P\"},\"type\":\"RecordBlkView.Signal\",\"uuid\":\"\"},{\"content\":{\"blockPath\":[],\"channel\":[2,4],\"dimensions\":[12,12],\"domain\":\"\",\"leafPath\":\"MATLAB System1:2.eresult.P\",\"lineColor\":\"#ff6929\",\"lineWidth\":2,\"parentID\":15,\"port\":1,\"sid\":[\"\"],\"signalID\":95,\"signalName\":\"MATLAB System1:2.eresult.P\"},\"type\":\"RecordBlkView.Signal\",\"uuid\":\"\"},{\"content\":{\"blockPath\":[],\"channel\":[3,4],\"dimensions\":[12,12],\"domain\":\"\",\"leafPath\":\"MATLAB System1:2.eresult.P\",\"lineColor\":\"#b746ff\",\"lineWidth\":2,\"parentID\":15,\"port\":1,\"sid\":[\"\"],\"signalID\":96,\"signalName\":\"MATLAB System1:2.eresult.P\"},\"type\":\"RecordBlkView.Signal\",\"uuid\":\"\"},{\"content\":{\"blockPath\":[],\"channel\":[4,4],\"dimensions\":[12,12],\"domain\":\"\",\"leafPath\":\"MATLAB System1:2.eresult.P\",\"lineColor\":\"#64d413\",\"lineWidth\":2,\"parentID\":15,\"port\":1,\"sid\":[\"\"],\"signalID\":97,\"signalName\":\"MATLAB System1:2.eresult.P\"},\"type\":\"RecordBlkView.Signal\",\"uuid\":\"\"},{\"content\":{\"blockPath\":[],\"channel\":[5,4],\"dimensions\":[12,12],\"domain\":\"\",\"leafPath\":\"MATLAB System1:2.eresult.P\",\"lineColor\":\"#ff13a6\",\"lineWidth\":2,\"parentID\":15,\"port\":1,\"sid\":[\"\"],\"signalID\":98,\"signalName\":\"MATLAB System1:2.eresult.P\"},\"type\":\"RecordBlkView.Signal\",\"uuid\":\"\"},{\"content\":{\"blockPath\":[],\"channel\":[6,4],\"dimensions\":[12,12],\"domain\":\"\",\"leafPath\":\"MATLAB System1:2.eresult.P\",\"lineColor\":\"#fe330a\",\"lineWidth\":2,\"parentID\":15,\"port\":1,\"sid\":[\"\"],\"signalID\":99,\"signalName\":\"MATLAB System1:2.eresult.P\"},\"type\":\"RecordBlkView.Signal\",\"uuid\":\"\"},{\"content\":{\"blockPath\":[],\"channel\":[7,4],\"dimensions\":[12,12],\"domain\":\"\",\"leafPath\":\"MATLAB System1:2.eresult.P\",\"lineColor\":\"#22b573\",\"lineWidth\":2,\"parentID\":15,\"port\":1,\"sid\":[\"\"],\"signalID\":100,\"signalName\":\"MATLAB System1:2.eresult.P\"},\"type\":\"RecordBlkView.Signal\",\"uuid\":\"\"},{\"content\":{\"blockPath\":[],\"channel\":[8,4],\"dimensions\":[12,12],\"domain\":\"\",\"leafPath\":\"MATLAB System1:2.eresult.P\",\"lineColor\":\"#0072bd\",\"lineWidth\":2,\"parentID\":15,\"port\":1,\"sid\":[\"\"],\"signalID\":101,\"signalName\":\"MATLAB System1:2.eresult.P\"},\"type\":\"RecordBlkView.Signal\",\"uuid\":\"\"},{\"content\":{\"blockPath\":[],\"channel\":[9,4],\"dimensions\":[12,12],\"domain\":\"\",\"leafPath\":\"MATLAB System1:2.eresult.P\",\"lineColor\":\"#d95319\",\"lineWidth\":2,\"parentID\":15,\"port\":1,\"sid\":[\"\"],\"signalID\":102,\"signalName\":\"MATLAB System1:2.eresult.P\"},\"type\":\"RecordBlkView.Signal\",\"uuid\":\"\"},{\"content\":{\"blockPath\":[],\"channel\":[10,4],\"dimensions\":[12,12],\"domain\":\"\",\"leafPath\":\"MATLAB System1:2.eresult.P\",\"lineColor\":\"#edb120\",\"lineWidth\":2,\"parentID\":15,\"port\":1,\"sid\":[\"\"],\"signalID\":103,\"signalName\":\"MATLAB System1:2.eresult.P\"},\"type\":\"RecordBlkView.Signal\",\"uuid\":\"\"},{\"content\":{\"blockPath\":[],\"channel\":[11,4],\"dimensions\":[12,12],\"domain\":\"\",\"leafPath\":\"MATLAB System1:2.eresult.P\",\"lineColor\":\"#7e2f8e\",\"lineWidth\":2,\"parentID\":15,\"port\":1,\"sid\":[\"\"],\"signalID\":104,\"signalName\":\"MATLAB System1:2.eresult.P\"},\"type\":\"RecordBlkView.Signal\",\"uuid\":\"\"},{\"content\":{\"blockPath\":[],\"channel\":[12,4],\"dimensions\":[12,12],\"domain\":\"\",\"leafPath\":\"MATLAB System1:2.eresult.P\",\"lineColor\":\"#77ac30\",\"lineWidth\":2,\"parentID\":15,\"port\":1,\"sid\":[\"\"],\"signalID\":105,\"signalName\":\"MATLAB System1:2.eresult.P\"},\"type\":\"RecordBlkView.Signal\",\"uuid\":\"\"},{\"content\":{\"blockPath\":[],\"channel\":[1,5],\"dimensions\":[12,12],\"domain\":\"\",\"leafPath\":\"MATLAB System1:2.eresult.P\",\"lineColor\":\"#4dbeee\",\"lineWidth\":2,\"parentID\":15,\"port\":1,\"sid\":[\"\"],\"signalID\":106,\"signalName\":\"MATLAB System1:2.eresult.P\"},\"type\":\"RecordBlkView.Signal\",\"uuid\":\"\"},{\"content\":{\"blockPath\":[],\"channel\":[2,5],\"dimensions\":[12,12],\"domain\":\"\",\"leafPath\":\"MATLAB System1:2.eresult.P\",\"lineColor\":\"#a2142f\",\"lineWidth\":2,\"parentID\":15,\"port\":1,\"sid\":[\"\"],\"signalID\":107,\"signalName\":\"MATLAB System1:2.eresult.P\"},\"type\":\"RecordBlkView.Signal\",\"uuid\":\"\"},{\"content\":{\"blockPath\":[],\"channel\":[3,5],\"dimensions\":[12,12],\"domain\":\"\",\"leafPath\":\"MATLAB System1:2.eresult.P\",\"lineColor\":\"#139fff\",\"lineWidth\":2,\"parentID\":15,\"port\":1,\"sid\":[\"\"],\"signalID\":108,\"signalName\":\"MATLAB System1:2.eresult.P\"},\"type\":\"RecordBlkView.Signal\",\"uuid\":\"\"},{\"content\":{\"blockPath\":[],\"channel\":[4,5],\"dimensions\":[12,12],\"domain\":\"\",\"leafPath\":\"MATLAB System1:2.eresult.P\",\"lineColor\":\"#ff6929\",\"lineWidth\":2,\"parentID\":15,\"port\":1,\"sid\":[\"\"],\"signalID\":109,\"signalName\":\"MATLAB System1:2.eresult.P\"},\"type\":\"RecordBlkView.Signal\",\"uuid\":\"\"},{\"content\":{\"blockPath\":[],\"channel\":[5,5],\"dimensions\":[12,12],\"domain\":\"\",\"leafPath\":\"MATLAB System1:2.eresult.P\",\"lineColor\":\"#b746ff\",\"lineWidth\":2,\"parentID\":15,\"port\":1,\"sid\":[\"\"],\"signalID\":110,\"signalName\":\"MATLAB System1:2.eresult.P\"},\"type\":\"RecordBlkView.Signal\",\"uuid\":\"\"},{\"content\":{\"blockPath\":[],\"channel\":[6,5],\"dimensions\":[12,12],\"domain\":\"\",\"leafPath\":\"MATLAB System1:2.eresult.P\",\"lineColor\":\"#64d413\",\"lineWidth\":2,\"parentID\":15,\"port\":1,\"sid\":[\"\"],\"signalID\":111,\"signalName\":\"MATLAB System1:2.eresult.P\"},\"type\":\"RecordBlkView.Signal\",\"uuid\":\"\"},{\"content\":{\"blockPath\":[],\"channel\":[7,5],\"dimensions\":[12,12],\"domain\":\"\",\"leafPath\":\"MATLAB System1:2.eresult.P\",\"lineColor\":\"#ff13a6\",\"lineWidth\":2,\"parentID\":15,\"port\":1,\"sid\":[\"\"],\"signalID\":112,\"signalName\":\"MATLAB System1:2.eresult.P\"},\"type\":\"RecordBlkView.Signal\",\"uuid\":\"\"},{\"content\":{\"blockPath\":[],\"channel\":[8,5],\"dimensions\":[12,12],\"domain\":\"\",\"leafPath\":\"MATLAB System1:2.eresult.P\",\"lineColor\":\"#fe330a\",\"lineWidth\":2,\"parentID\":15,\"port\":1,\"sid\":[\"\"],\"signalID\":113,\"signalName\":\"MATLAB System1:2.eresult.P\"},\"type\":\"RecordBlkView.Signal\",\"uuid\":\"\"},{\"content\":{\"blockPath\":[],\"channel\":[9,5],\"dimensions\":[12,12],\"domain\":\"\",\"leafPath\":\"MATLAB System1:2.eresult.P\",\"lineColor\":\"#22b573\",\"lineWidth\":2,\"parentID\":15,\"port\":1,\"sid\":[\"\"],\"signalID\":114,\"signalName\":\"MATLAB System1:2.eresult.P\"},\"type\":\"RecordBlkView.Signal\",\"uuid\":\"\"},{\"content\":{\"blockPath\":[],\"channel\":[10,5],\"dimensions\":[12,12],\"domain\":\"\",\"leafPath\":\"MATLAB System1:2.eresult.P\",\"lineColor\":\"#0072bd\",\"lineWidth\":2,\"parentID\":15,\"port\":1,\"sid\":[\"\"],\"signalID\":115,\"signalName\":\"MATLAB System1:2.eresult.P\"},\"type\":\"RecordBlkView.Signal\",\"uuid\":\"\"},{\"content\":{\"blockPath\":[],\"channel\":[11,5],\"dimensions\":[12,12],\"domain\":\"\",\"leafPath\":\"MATLAB System1:2.eresult.P\",\"lineColor\":\"#d95319\",\"lineWidth\":2,\"parentID\":15,\"port\":1,\"sid\":[\"\"],\"signalID\":116,\"signalName\":\"MATLAB System1:2.eresult.P\"},\"type\":\"RecordBlkView.Signal\",\"uuid\":\"\"},{\"content\":{\"blockPath\":[],\"channel\":[12,5],\"dimensions\":[12,12],\"domain\":\"\",\"leafPath\":\"MATLAB System1:2.eresult.P\",\"lineColor\":\"#edb120\",\"lineWidth\":2,\"parentID\":15,\"port\":1,\"sid\":[\"\"],\"signalID\":117,\"signalName\":\"MATLAB System1:2.eresult.P\"},\"type\":\"RecordBlkView.Signal\",\"uuid\":\"\"},{\"content\":{\"blockPath\":[],\"channel\":[1,6],\"dimensions\":[12,12],\"domain\":\"\",\"leafPath\":\"MATLAB System1:2.eresult.P\",\"lineColor\":\"#7e2f8e\",\"lineWidth\":2,\"parentID\":15,\"port\":1,\"sid\":[\"\"],\"signalID\":118,\"signalName\":\"MATLAB System1:2.eresult.P\"},\"type\":\"RecordBlkView.Signal\",\"uuid\":\"\"},{\"content\":{\"blockPath\":[],\"channel\":[2,6],\"dimensions\":[12,12],\"domain\":\"\",\"leafPath\":\"MATLAB System1:2.eresult.P\",\"lineColor\":\"#77ac30\",\"lineWidth\":2,\"parentID\":15,\"port\":1,\"sid\":[\"\"],\"signalID\":119,\"signalName\":\"MATLAB System1:2.eresult.P\"},\"type\":\"RecordBlkView.Signal\",\"uuid\":\"\"},{\"content\":{\"blockPath\":[],\"channel\":[3,6],\"dimensions\":[12,12],\"domain\":\"\",\"leafPath\":\"MATLAB System1:2.eresult.P\",\"lineColor\":\"#4dbeee\",\"lineWidth\":2,\"parentID\":15,\"port\":1,\"sid\":[\"\"],\"signalID\":120,\"signalName\":\"MATLAB System1:2.eresult.P\"},\"type\":\"RecordBlkView.Signal\",\"uuid\":\"\"},{\"content\":{\"blockPath\":[],\"channel\":[4,6],\"dimensions\":[12,12],\"domain\":\"\",\"leafPath\":\"MATLAB System1:2.eresult.P\",\"lineColor\":\"#a2142f\",\"lineWidth\":2,\"parentID\":15,\"port\":1,\"sid\":[\"\"],\"signalID\":121,\"signalName\":\"MATLAB System1:2.eresult.P\"},\"type\":\"RecordBlkView.Signal\",\"uuid\":\"\"},{\"content\":{\"blockPath\":[],\"channel\":[5,6],\"dimensions\":[12,12],\"domain\":\"\",\"leafPath\":\"MATLAB System1:2.eresult.P\",\"lineColor\":\"#139fff\",\"lineWidth\":2,\"parentID\":15,\"port\":1,\"sid\":[\"\"],\"signalID\":122,\"signalName\":\"MATLAB System1:2.eresult.P\"},\"type\":\"RecordBlkView.Signal\",\"uuid\":\"\"},{\"content\":{\"blockPath\":[],\"channel\":[6,6],\"dimensions\":[12,12],\"domain\":\"\",\"leafPath\":\"MATLAB System1:2.eresult.P\",\"lineColor\":\"#ff6929\",\"lineWidth\":2,\"parentID\":15,\"port\":1,\"sid\":[\"\"],\"signalID\":123,\"signalName\":\"MATLAB System1:2.eresult.P\"},\"type\":\"RecordBlkView.Signal\",\"uuid\":\"\"},{\"content\":{\"blockPath\":[],\"channel\":[7,6],\"dimensions\":[12,12],\"domain\":\"\",\"leafPath\":\"MATLAB System1:2.eresult.P\",\"lineColor\":\"#b746ff\",\"lineWidth\":2,\"parentID\":15,\"port\":1,\"sid\":[\"\"],\"signalID\":124,\"signalName\":\"MATLAB System1:2.eresult.P\"},\"type\":\"RecordBlkView.Signal\",\"uuid\":\"\"},{\"content\":{\"blockPath\":[],\"channel\":[8,6],\"dimensions\":[12,12],\"domain\":\"\",\"leafPath\":\"MATLAB System1:2.eresult.P\",\"lineColor\":\"#64d413\",\"lineWidth\":2,\"parentID\":15,\"port\":1,\"sid\":[\"\"],\"signalID\":125,\"signalName\":\"MATLAB System1:2.eresult.P\"},\"type\":\"RecordBlkView.Signal\",\"uuid\":\"\"},{\"content\":{\"blockPath\":[],\"channel\":[9,6],\"dimensions\":[12,12],\"domain\":\"\",\"leafPath\":\"MATLAB System1:2.eresult.P\",\"lineColor\":\"#ff13a6\",\"lineWidth\":2,\"parentID\":15,\"port\":1,\"sid\":[\"\"],\"signalID\":126,\"signalName\":\"MATLAB System1:2.eresult.P\"},\"type\":\"RecordBlkView.Signal\",\"uuid\":\"\"},{\"content\":{\"blockPath\":[],\"channel\":[10,6],\"dimensions\":[12,12],\"domain\":\"\",\"leafPath\":\"MATLAB System1:2.eresult.P\",\"lineColor\":\"#fe330a\",\"lineWidth\":2,\"parentID\":15,\"port\":1,\"sid\":[\"\"],\"signalID\":127,\"signalName\":\"MATLAB System1:2.eresult.P\"},\"type\":\"RecordBlkView.Signal\",\"uuid\":\"\"},{\"content\":{\"blockPath\":[],\"channel\":[11,6],\"dimensions\":[12,12],\"domain\":\"\",\"leafPath\":\"MATLAB System1:2.eresult.P\",\"lineColor\":\"#22b573\",\"lineWidth\":2,\"parentID\":15,\"port\":1,\"sid\":[\"\"],\"signalID\":128,\"signalName\":\"MATLAB System1:2.eresult.P\"},\"type\":\"RecordBlkView.Signal\",\"uuid\":\"\"},{\"content\":{\"blockPath\":[],\"channel\":[12,6],\"dimensions\":[12,12],\"domain\":\"\",\"leafPath\":\"MATLAB System1:2.eresult.P\",\"lineColor\":\"#0072bd\",\"lineWidth\":2,\"parentID\":15,\"port\":1,\"sid\":[\"\"],\"signalID\":129,\"signalName\":\"MATLAB System1:2.eresult.P\"},\"type\":\"RecordBlkView.Signal\",\"uuid\":\"\"},{\"content\":{\"blockPath\":[],\"channel\":[1,7],\"dimensions\":[12,12],\"domain\":\"\",\"leafPath\":\"MATLAB System1:2.eresult.P\",\"lineColor\":\"#d95319\",\"lineWidth\":2,\"parentID\":15,\"port\":1,\"sid\":[\"\"],\"signalID\":130,\"signalName\":\"MATLAB System1:2.eresult.P\"},\"type\":\"RecordBlkView.Signal\",\"uuid\":\"\"},{\"content\":{\"blockPath\":[],\"channel\":[2,7],\"dimensions\":[12,12],\"domain\":\"\",\"leafPath\":\"MATLAB System1:2.eresult.P\",\"lineColor\":\"#edb120\",\"lineWidth\":2,\"parentID\":15,\"port\":1,\"sid\":[\"\"],\"signalID\":131,\"signalName\":\"MATLAB System1:2.eresult.P\"},\"type\":\"RecordBlkView.Signal\",\"uuid\":\"\"},{\"content\":{\"blockPath\":[],\"channel\":[3,7],\"dimensions\":[12,12],\"domain\":\"\",\"leafPath\":\"MATLAB System1:2.eresult.P\",\"lineColor\":\"#7e2f8e\",\"lineWidth\":2,\"parentID\":15,\"port\":1,\"sid\":[\"\"],\"signalID\":132,\"signalName\":\"MATLAB System1:2.eresult.P\"},\"type\":\"RecordBlkView.Signal\",\"uuid\":\"\"},{\"content\":{\"blockPath\":[],\"channel\":[4,7],\"dimensions\":[12,12],\"domain\":\"\",\"leafPath\":\"MATLAB System1:2.eresult.P\",\"lineColor\":\"#77ac30\",\"lineWidth\":2,\"parentID\":15,\"port\":1,\"sid\":[\"\"],\"signalID\":133,\"signalName\":\"MATLAB System1:2.eresult.P\"},\"type\":\"RecordBlkView.Signal\",\"uuid\":\"\"},{\"content\":{\"blockPath\":[],\"channel\":[5,7],\"dimensions\":[12,12],\"domain\":\"\",\"leafPath\":\"MATLAB System1:2.eresult.P\",\"lineColor\":\"#4dbeee\",\"lineWidth\":2,\"parentID\":15,\"port\":1,\"sid\":[\"\"],\"signalID\":134,\"signalName\":\"MATLAB System1:2.eresult.P\"},\"type\":\"RecordBlkView.Signal\",\"uuid\":\"\"},{\"content\":{\"blockPath\":[],\"channel\":[6,7],\"dimensions\":[12,12],\"domain\":\"\",\"leafPath\":\"MATLAB System1:2.eresult.P\",\"lineColor\":\"#a2142f\",\"lineWidth\":2,\"parentID\":15,\"port\":1,\"sid\":[\"\"],\"signalID\":135,\"signalName\":\"MATLAB System1:2.eresult.P\"},\"type\":\"RecordBlkView.Signal\",\"uuid\":\"\"},{\"content\":{\"blockPath\":[],\"channel\":[7,7],\"dimensions\":[12,12],\"domain\":\"\",\"leafPath\":\"MATLAB System1:2.eresult.P\",\"lineColor\":\"#139fff\",\"lineWidth\":2,\"parentID\":15,\"port\":1,\"sid\":[\"\"],\"signalID\":136,\"signalName\":\"MATLAB System1:2.eresult.P\"},\"type\":\"RecordBlkView.Signal\",\"uuid\":\"\"},{\"content\":{\"blockPath\":[],\"channel\":[8,7],\"dimensions\":[12,12],\"domain\":\"\",\"leafPath\":\"MATLAB System1:2.eresult.P\",\"lineColor\":\"#ff6929\",\"lineWidth\":2,\"parentID\":15,\"port\":1,\"sid\":[\"\"],\"signalID\":137,\"signalName\":\"MATLAB System1:2.eresult.P\"},\"type\":\"RecordBlkView.Signal\",\"uuid\":\"\"},{\"content\":{\"blockPath\":[],\"channel\":[9,7],\"dimensions\":[12,12],\"domain\":\"\",\"leafPath\":\"MATLAB System1:2.eresult.P\",\"lineColor\":\"#b746ff\",\"lineWidth\":2,\"parentID\":15,\"port\":1,\"sid\":[\"\"],\"signalID\":138,\"signalName\":\"MATLAB System1:2.eresult.P\"},\"type\":\"RecordBlkView.Signal\",\"uuid\":\"\"},{\"content\":{\"blockPath\":[],\"channel\":[10,7],\"dimensions\":[12,12],\"domain\":\"\",\"leafPath\":\"MATLAB System1:2.eresult.P\",\"lineColor\":\"#64d413\",\"lineWidth\":2,\"parentID\":15,\"port\":1,\"sid\":[\"\"],\"signalID\":139,\"signalName\":\"MATLAB System1:2.eresult.P\"},\"type\":\"RecordBlkView.Signal\",\"uuid\":\"\"},{\"content\":{\"blockPath\":[],\"channel\":[11,7],\"dimensions\":[12,12],\"domain\":\"\",\"leafPath\":\"MATLAB System1:2.eresult.P\",\"lineColor\":\"#ff13a6\",\"lineWidth\":2,\"parentID\":15,\"port\":1,\"sid\":[\"\"],\"signalID\":140,\"signalName\":\"MATLAB System1:2.eresult.P\"},\"type\":\"RecordBlkView.Signal\",\"uuid\":\"\"},{\"content\":{\"blockPath\":[],\"channel\":[12,7],\"dimensions\":[12,12],\"domain\":\"\",\"leafPath\":\"MATLAB System1:2.eresult.P\",\"lineColor\":\"#fe330a\",\"lineWidth\":2,\"parentID\":15,\"port\":1,\"sid\":[\"\"],\"signalID\":141,\"signalName\":\"MATLAB System1:2.eresult.P\"},\"type\":\"RecordBlkView.Signal\",\"uuid\":\"\"},{\"content\":{\"blockPath\":[],\"channel\":[1,8],\"dimensions\":[12,12],\"domain\":\"\",\"leafPath\":\"MATLAB System1:2.eresult.P\",\"lineColor\":\"#22b573\",\"lineWidth\":2,\"parentID\":15,\"port\":1,\"sid\":[\"\"],\"signalID\":142,\"signalName\":\"MATLAB System1:2.eresult.P\"},\"type\":\"RecordBlkView.Signal\",\"uuid\":\"\"},{\"content\":{\"blockPath\":[],\"channel\":[2,8],\"dimensions\":[12,12],\"domain\":\"\",\"leafPath\":\"MATLAB System1:2.eresult.P\",\"lineColor\":\"#0072bd\",\"lineWidth\":2,\"parentID\":15,\"port\":1,\"sid\":[\"\"],\"signalID\":143,\"signalName\":\"MATLAB System1:2.eresult.P\"},\"type\":\"RecordBlkView.Signal\",\"uuid\":\"\"},{\"content\":{\"blockPath\":[],\"channel\":[3,8],\"dimensions\":[12,12],\"domain\":\"\",\"leafPath\":\"MATLAB System1:2.eresult.P\",\"lineColor\":\"#d95319\",\"lineWidth\":2,\"parentID\":15,\"port\":1,\"sid\":[\"\"],\"signalID\":144,\"signalName\":\"MATLAB System1:2.eresult.P\"},\"type\":\"RecordBlkView.Signal\",\"uuid\":\"\"},{\"content\":{\"blockPath\":[],\"channel\":[4,8],\"dimensions\":[12,12],\"domain\":\"\",\"leafPath\":\"MATLAB System1:2.eresult.P\",\"lineColor\":\"#edb120\",\"lineWidth\":2,\"parentID\":15,\"port\":1,\"sid\":[\"\"],\"signalID\":145,\"signalName\":\"MATLAB System1:2.eresult.P\"},\"type\":\"RecordBlkView.Signal\",\"uuid\":\"\"},{\"content\":{\"blockPath\":[],\"channel\":[5,8],\"dimensions\":[12,12],\"domain\":\"\",\"leafPath\":\"MATLAB System1:2.eresult.P\",\"lineColor\":\"#7e2f8e\",\"lineWidth\":2,\"parentID\":15,\"port\":1,\"sid\":[\"\"],\"signalID\":146,\"signalName\":\"MATLAB System1:2.eresult.P\"},\"type\":\"RecordBlkView.Signal\",\"uuid\":\"\"},{\"content\":{\"blockPath\":[],\"channel\":[6,8],\"dimensions\":[12,12],\"domain\":\"\",\"leafPath\":\"MATLAB System1:2.eresult.P\",\"lineColor\":\"#77ac30\",\"lineWidth\":2,\"parentID\":15,\"port\":1,\"sid\":[\"\"],\"signalID\":147,\"signalName\":\"MATLAB System1:2.eresult.P\"},\"type\":\"RecordBlkView.Signal\",\"uuid\":\"\"},{\"content\":{\"blockPath\":[],\"channel\":[7,8],\"dimensions\":[12,12],\"domain\":\"\",\"leafPath\":\"MATLAB System1:2.eresult.P\",\"lineColor\":\"#4dbeee\",\"lineWidth\":2,\"parentID\":15,\"port\":1,\"sid\":[\"\"],\"signalID\":148,\"signalName\":\"MATLAB System1:2.eresult.P\"},\"type\":\"RecordBlkView.Signal\",\"uuid\":\"\"},{\"content\":{\"blockPath\":[],\"channel\":[8,8],\"dimensions\":[12,12],\"domain\":\"\",\"leafPath\":\"MATLAB System1:2.eresult.P\",\"lineColor\":\"#a2142f\",\"lineWidth\":2,\"parentID\":15,\"port\":1,\"sid\":[\"\"],\"signalID\":149,\"signalName\":\"MATLAB System1:2.eresult.P\"},\"type\":\"RecordBlkView.Signal\",\"uuid\":\"\"},{\"content\":{\"blockPath\":[],\"channel\":[9,8],\"dimensions\":[12,12],\"domain\":\"\",\"leafPath\":\"MATLAB System1:2.eresult.P\",\"lineColor\":\"#139fff\",\"lineWidth\":2,\"parentID\":15,\"port\":1,\"sid\":[\"\"],\"signalID\":150,\"signalName\":\"MATLAB System1:2.eresult.P\"},\"type\":\"RecordBlkView.Signal\",\"uuid\":\"\"},{\"content\":{\"blockPath\":[],\"channel\":[10,8],\"dimensions\":[12,12],\"domain\":\"\",\"leafPath\":\"MATLAB System1:2.eresult.P\",\"lineColor\":\"#ff6929\",\"lineWidth\":2,\"parentID\":15,\"port\":1,\"sid\":[\"\"],\"signalID\":151,\"signalName\":\"MATLAB System1:2.eresult.P\"},\"type\":\"RecordBlkView.Signal\",\"uuid\":\"\"},{\"content\":{\"blockPath\":[],\"channel\":[11,8],\"dimensions\":[12,12],\"domain\":\"\",\"leafPath\":\"MATLAB System1:2.eresult.P\",\"lineColor\":\"#b746ff\",\"lineWidth\":2,\"parentID\":15,\"port\":1,\"sid\":[\"\"],\"signalID\":152,\"signalName\":\"MATLAB System1:2.eresult.P\"},\"type\":\"RecordBlkView.Signal\",\"uuid\":\"\"},{\"content\":{\"blockPath\":[],\"channel\":[12,8],\"dimensions\":[12,12],\"domain\":\"\",\"leafPath\":\"MATLAB System1:2.eresult.P\",\"lineColor\":\"#64d413\",\"lineWidth\":2,\"parentID\":15,\"port\":1,\"sid\":[\"\"],\"signalID\":153,\"signalName\":\"MATLAB System1:2.eresult.P\"},\"type\":\"RecordBlkView.Signal\",\"uuid\":\"\"},{\"content\":{\"blockPath\":[],\"channel\":[1,9],\"dimensions\":[12,12],\"domain\":\"\",\"leafPath\":\"MATLAB System1:2.eresult.P\",\"lineColor\":\"#ff13a6\",\"lineWidth\":2,\"parentID\":15,\"port\":1,\"sid\":[\"\"],\"signalID\":154,\"signalName\":\"MATLAB System1:2.eresult.P\"},\"type\":\"RecordBlkView.Signal\",\"uuid\":\"\"},{\"content\":{\"blockPath\":[],\"channel\":[2,9],\"dimensions\":[12,12],\"domain\":\"\",\"leafPath\":\"MATLAB System1:2.eresult.P\",\"lineColor\":\"#fe330a\",\"lineWidth\":2,\"parentID\":15,\"port\":1,\"sid\":[\"\"],\"signalID\":155,\"signalName\":\"MATLAB System1:2.eresult.P\"},\"type\":\"RecordBlkView.Signal\",\"uuid\":\"\"},{\"content\":{\"blockPath\":[],\"channel\":[3,9],\"dimensions\":[12,12],\"domain\":\"\",\"leafPath\":\"MATLAB System1:2.eresult.P\",\"lineColor\":\"#22b573\",\"lineWidth\":2,\"parentID\":15,\"port\":1,\"sid\":[\"\"],\"signalID\":156,\"signalName\":\"MATLAB System1:2.eresult.P\"},\"type\":\"RecordBlkView.Signal\",\"uuid\":\"\"},{\"content\":{\"blockPath\":[],\"channel\":[4,9],\"dimensions\":[12,12],\"domain\":\"\",\"leafPath\":\"MATLAB System1:2.eresult.P\",\"lineColor\":\"#0072bd\",\"lineWidth\":2,\"parentID\":15,\"port\":1,\"sid\":[\"\"],\"signalID\":157,\"signalName\":\"MATLAB System1:2.eresult.P\"},\"type\":\"RecordBlkView.Signal\",\"uuid\":\"\"},{\"content\":{\"blockPath\":[],\"channel\":[5,9],\"dimensions\":[12,12],\"domain\":\"\",\"leafPath\":\"MATLAB System1:2.eresult.P\",\"lineColor\":\"#d95319\",\"lineWidth\":2,\"parentID\":15,\"port\":1,\"sid\":[\"\"],\"signalID\":158,\"signalName\":\"MATLAB System1:2.eresult.P\"},\"type\":\"RecordBlkView.Signal\",\"uuid\":\"\"},{\"content\":{\"blockPath\":[],\"channel\":[6,9],\"dimensions\":[12,12],\"domain\":\"\",\"leafPath\":\"MATLAB System1:2.eresult.P\",\"lineColor\":\"#edb120\",\"lineWidth\":2,\"parentID\":15,\"port\":1,\"sid\":[\"\"],\"signalID\":159,\"signalName\":\"MATLAB System1:2.eresult.P\"},\"type\":\"RecordBlkView.Signal\",\"uuid\":\"\"},{\"content\":{\"blockPath\":[],\"channel\":[7,9],\"dimensions\":[12,12],\"domain\":\"\",\"leafPath\":\"MATLAB System1:2.eresult.P\",\"lineColor\":\"#7e2f8e\",\"lineWidth\":2,\"parentID\":15,\"port\":1,\"sid\":[\"\"],\"signalID\":160,\"signalName\":\"MATLAB System1:2.eresult.P\"},\"type\":\"RecordBlkView.Signal\",\"uuid\":\"\"},{\"content\":{\"blockPath\":[],\"channel\":[8,9],\"dimensions\":[12,12],\"domain\":\"\",\"leafPath\":\"MATLAB System1:2.eresult.P\",\"lineColor\":\"#77ac30\",\"lineWidth\":2,\"parentID\":15,\"port\":1,\"sid\":[\"\"],\"signalID\":161,\"signalName\":\"MATLAB System1:2.eresult.P\"},\"type\":\"RecordBlkView.Signal\",\"uuid\":\"\"},{\"content\":{\"blockPath\":[],\"channel\":[9,9],\"dimensions\":[12,12],\"domain\":\"\",\"leafPath\":\"MATLAB System1:2.eresult.P\",\"lineColor\":\"#4dbeee\",\"lineWidth\":2,\"parentID\":15,\"port\":1,\"sid\":[\"\"],\"signalID\":162,\"signalName\":\"MATLAB System1:2.eresult.P\"},\"type\":\"RecordBlkView.Signal\",\"uuid\":\"\"},{\"content\":{\"blockPath\":[],\"channel\":[10,9],\"dimensions\":[12,12],\"domain\":\"\",\"leafPath\":\"MATLAB System1:2.eresult.P\",\"lineColor\":\"#a2142f\",\"lineWidth\":2,\"parentID\":15,\"port\":1,\"sid\":[\"\"],\"signalID\":163,\"signalName\":\"MATLAB System1:2.eresult.P\"},\"type\":\"RecordBlkView.Signal\",\"uuid\":\"\"},{\"content\":{\"blockPath\":[],\"channel\":[11,9],\"dimensions\":[12,12],\"domain\":\"\",\"leafPath\":\"MATLAB System1:2.eresult.P\",\"lineColor\":\"#139fff\",\"lineWidth\":2,\"parentID\":15,\"port\":1,\"sid\":[\"\"],\"signalID\":164,\"signalName\":\"MATLAB System1:2.eresult.P\"},\"type\":\"RecordBlkView.Signal\",\"uuid\":\"\"},{\"content\":{\"blockPath\":[],\"channel\":[12,9],\"dimensions\":[12,12],\"domain\":\"\",\"leafPath\":\"MATLAB System1:2.eresult.P\",\"lineColor\":\"#ff6929\",\"lineWidth\":2,\"parentID\":15,\"port\":1,\"sid\":[\"\"],\"signalID\":165,\"signalName\":\"MATLAB System1:2.eresult.P\"},\"type\":\"RecordBlkView.Signal\",\"uuid\":\"\"},{\"content\":{\"blockPath\":[],\"channel\":[1,10],\"dimensions\":[12,12],\"domain\":\"\",\"leafPath\":\"MATLAB System1:2.eresult.P\",\"lineColor\":\"#b746ff\",\"lineWidth\":2,\"parentID\":15,\"port\":1,\"sid\":[\"\"],\"signalID\":166,\"signalName\":\"MATLAB System1:2.eresult.P\"},\"type\":\"RecordBlkView.Signal\",\"uuid\":\"\"},{\"content\":{\"blockPath\":[],\"channel\":[2,10],\"dimensions\":[12,12],\"domain\":\"\",\"leafPath\":\"MATLAB System1:2.eresult.P\",\"lineColor\":\"#64d413\",\"lineWidth\":2,\"parentID\":15,\"port\":1,\"sid\":[\"\"],\"signalID\":167,\"signalName\":\"MATLAB System1:2.eresult.P\"},\"type\":\"RecordBlkView.Signal\",\"uuid\":\"\"},{\"content\":{\"blockPath\":[],\"channel\":[3,10],\"dimensions\":[12,12],\"domain\":\"\",\"leafPath\":\"MATLAB System1:2.eresult.P\",\"lineColor\":\"#ff13a6\",\"lineWidth\":2,\"parentID\":15,\"port\":1,\"sid\":[\"\"],\"signalID\":168,\"signalName\":\"MATLAB System1:2.eresult.P\"},\"type\":\"RecordBlkView.Signal\",\"uuid\":\"\"},{\"content\":{\"blockPath\":[],\"channel\":[4,10],\"dimensions\":[12,12],\"domain\":\"\",\"leafPath\":\"MATLAB System1:2.eresult.P\",\"lineColor\":\"#fe330a\",\"lineWidth\":2,\"parentID\":15,\"port\":1,\"sid\":[\"\"],\"signalID\":169,\"signalName\":\"MATLAB System1:2.eresult.P\"},\"type\":\"RecordBlkView.Signal\",\"uuid\":\"\"},{\"content\":{\"blockPath\":[],\"channel\":[5,10],\"dimensions\":[12,12],\"domain\":\"\",\"leafPath\":\"MATLAB System1:2.eresult.P\",\"lineColor\":\"#22b573\",\"lineWidth\":2,\"parentID\":15,\"port\":1,\"sid\":[\"\"],\"signalID\":170,\"signalName\":\"MATLAB System1:2.eresult.P\"},\"type\":\"RecordBlkView.Signal\",\"uuid\":\"\"},{\"content\":{\"blockPath\":[],\"channel\":[6,10],\"dimensions\":[12,12],\"domain\":\"\",\"leafPath\":\"MATLAB System1:2.eresult.P\",\"lineColor\":\"#0072bd\",\"lineWidth\":2,\"parentID\":15,\"port\":1,\"sid\":[\"\"],\"signalID\":171,\"signalName\":\"MATLAB System1:2.eresult.P\"},\"type\":\"RecordBlkView.Signal\",\"uuid\":\"\"},{\"content\":{\"blockPath\":[],\"channel\":[7,10],\"dimensions\":[12,12],\"domain\":\"\",\"leafPath\":\"MATLAB System1:2.eresult.P\",\"lineColor\":\"#d95319\",\"lineWidth\":2,\"parentID\":15,\"port\":1,\"sid\":[\"\"],\"signalID\":172,\"signalName\":\"MATLAB System1:2.eresult.P\"},\"type\":\"RecordBlkView.Signal\",\"uuid\":\"\"},{\"content\":{\"blockPath\":[],\"channel\":[8,10],\"dimensions\":[12,12],\"domain\":\"\",\"leafPath\":\"MATLAB System1:2.eresult.P\",\"lineColor\":\"#edb120\",\"lineWidth\":2,\"parentID\":15,\"port\":1,\"sid\":[\"\"],\"signalID\":173,\"signalName\":\"MATLAB System1:2.eresult.P\"},\"type\":\"RecordBlkView.Signal\",\"uuid\":\"\"},{\"content\":{\"blockPath\":[],\"channel\":[9,10],\"dimensions\":[12,12],\"domain\":\"\",\"leafPath\":\"MATLAB System1:2.eresult.P\",\"lineColor\":\"#7e2f8e\",\"lineWidth\":2,\"parentID\":15,\"port\":1,\"sid\":[\"\"],\"signalID\":174,\"signalName\":\"MATLAB System1:2.eresult.P\"},\"type\":\"RecordBlkView.Signal\",\"uuid\":\"\"},{\"content\":{\"blockPath\":[],\"channel\":[10,10],\"dimensions\":[12,12],\"domain\":\"\",\"leafPath\":\"MATLAB System1:2.eresult.P\",\"lineColor\":\"#77ac30\",\"lineWidth\":2,\"parentID\":15,\"port\":1,\"sid\":[\"\"],\"signalID\":175,\"signalName\":\"MATLAB System1:2.eresult.P\"},\"type\":\"RecordBlkView.Signal\",\"uuid\":\"\"},{\"content\":{\"blockPath\":[],\"channel\":[11,10],\"dimensions\":[12,12],\"domain\":\"\",\"leafPath\":\"MATLAB System1:2.eresult.P\",\"lineColor\":\"#4dbeee\",\"lineWidth\":2,\"parentID\":15,\"port\":1,\"sid\":[\"\"],\"signalID\":176,\"signalName\":\"MATLAB System1:2.eresult.P\"},\"type\":\"RecordBlkView.Signal\",\"uuid\":\"\"},{\"content\":{\"blockPath\":[],\"channel\":[12,10],\"dimensions\":[12,12],\"domain\":\"\",\"leafPath\":\"MATLAB System1:2.eresult.P\",\"lineColor\":\"#a2142f\",\"lineWidth\":2,\"parentID\":15,\"port\":1,\"sid\":[\"\"],\"signalID\":177,\"signalName\":\"MATLAB System1:2.eresult.P\"},\"type\":\"RecordBlkView.Signal\",\"uuid\":\"\"},{\"content\":{\"blockPath\":[],\"channel\":[1,11],\"dimensions\":[12,12],\"domain\":\"\",\"leafPath\":\"MATLAB System1:2.eresult.P\",\"lineColor\":\"#139fff\",\"lineWidth\":2,\"parentID\":15,\"port\":1,\"sid\":[\"\"],\"signalID\":178,\"signalName\":\"MATLAB System1:2.eresult.P\"},\"type\":\"RecordBlkView.Signal\",\"uuid\":\"\"},{\"content\":{\"blockPath\":[],\"channel\":[2,11],\"dimensions\":[12,12],\"domain\":\"\",\"leafPath\":\"MATLAB System1:2.eresult.P\",\"lineColor\":\"#ff6929\",\"lineWidth\":2,\"parentID\":15,\"port\":1,\"sid\":[\"\"],\"signalID\":179,\"signalName\":\"MATLAB System1:2.eresult.P\"},\"type\":\"RecordBlkView.Signal\",\"uuid\":\"\"},{\"content\":{\"blockPath\":[],\"channel\":[3,11],\"dimensions\":[12,12],\"domain\":\"\",\"leafPath\":\"MATLAB System1:2.eresult.P\",\"lineColor\":\"#b746ff\",\"lineWidth\":2,\"parentID\":15,\"port\":1,\"sid\":[\"\"],\"signalID\":180,\"signalName\":\"MATLAB System1:2.eresult.P\"},\"type\":\"RecordBlkView.Signal\",\"uuid\":\"\"},{\"content\":{\"blockPath\":[],\"channel\":[4,11],\"dimensions\":[12,12],\"domain\":\"\",\"leafPath\":\"MATLAB System1:2.eresult.P\",\"lineColor\":\"#64d413\",\"lineWidth\":2,\"parentID\":15,\"port\":1,\"sid\":[\"\"],\"signalID\":181,\"signalName\":\"MATLAB System1:2.eresult.P\"},\"type\":\"RecordBlkView.Signal\",\"uuid\":\"\"},{\"content\":{\"blockPath\":[],\"channel\":[5,11],\"dimensions\":[12,12],\"domain\":\"\",\"leafPath\":\"MATLAB System1:2.eresult.P\",\"lineColor\":\"#ff13a6\",\"lineWidth\":2,\"parentID\":15,\"port\":1,\"sid\":[\"\"],\"signalID\":182,\"signalName\":\"MATLAB System1:2.eresult.P\"},\"type\":\"RecordBlkView.Signal\",\"uuid\":\"\"},{\"content\":{\"blockPath\":[],\"channel\":[6,11],\"dimensions\":[12,12],\"domain\":\"\",\"leafPath\":\"MATLAB System1:2.eresult.P\",\"lineColor\":\"#fe330a\",\"lineWidth\":2,\"parentID\":15,\"port\":1,\"sid\":[\"\"],\"signalID\":183,\"signalName\":\"MATLAB System1:2.eresult.P\"},\"type\":\"RecordBlkView.Signal\",\"uuid\":\"\"},{\"content\":{\"blockPath\":[],\"channel\":[7,11],\"dimensions\":[12,12],\"domain\":\"\",\"leafPath\":\"MATLAB System1:2.eresult.P\",\"lineColor\":\"#22b573\",\"lineWidth\":2,\"parentID\":15,\"port\":1,\"sid\":[\"\"],\"signalID\":184,\"signalName\":\"MATLAB System1:2.eresult.P\"},\"type\":\"RecordBlkView.Signal\",\"uuid\":\"\"},{\"content\":{\"blockPath\":[],\"channel\":[8,11],\"dimensions\":[12,12],\"domain\":\"\",\"leafPath\":\"MATLAB System1:2.eresult.P\",\"lineColor\":\"#0072bd\",\"lineWidth\":2,\"parentID\":15,\"port\":1,\"sid\":[\"\"],\"signalID\":185,\"signalName\":\"MATLAB System1:2.eresult.P\"},\"type\":\"RecordBlkView.Signal\",\"uuid\":\"\"},{\"content\":{\"blockPath\":[],\"channel\":[9,11],\"dimensions\":[12,12],\"domain\":\"\",\"leafPath\":\"MATLAB System1:2.eresult.P\",\"lineColor\":\"#d95319\",\"lineWidth\":2,\"parentID\":15,\"port\":1,\"sid\":[\"\"],\"signalID\":186,\"signalName\":\"MATLAB System1:2.eresult.P\"},\"type\":\"RecordBlkView.Signal\",\"uuid\":\"\"},{\"content\":{\"blockPath\":[],\"channel\":[10,11],\"dimensions\":[12,12],\"domain\":\"\",\"leafPath\":\"MATLAB System1:2.eresult.P\",\"lineColor\":\"#edb120\",\"lineWidth\":2,\"parentID\":15,\"port\":1,\"sid\":[\"\"],\"signalID\":187,\"signalName\":\"MATLAB System1:2.eresult.P\"},\"type\":\"RecordBlkView.Signal\",\"uuid\":\"\"},{\"content\":{\"blockPath\":[],\"channel\":[11,11],\"dimensions\":[12,12],\"domain\":\"\",\"leafPath\":\"MATLAB System1:2.eresult.P\",\"lineColor\":\"#7e2f8e\",\"lineWidth\":2,\"parentID\":15,\"port\":1,\"sid\":[\"\"],\"signalID\":188,\"signalName\":\"MATLAB System1:2.eresult.P\"},\"type\":\"RecordBlkView.Signal\",\"uuid\":\"\"},{\"content\":{\"blockPath\":[],\"channel\":[12,11],\"dimensions\":[12,12],\"domain\":\"\",\"leafPath\":\"MATLAB System1:2.eresult.P\",\"lineColor\":\"#77ac30\",\"lineWidth\":2,\"parentID\":15,\"port\":1,\"sid\":[\"\"],\"signalID\":189,\"signalName\":\"MATLAB System1:2.eresult.P\"},\"type\":\"RecordBlkView.Signal\",\"uuid\":\"\"},{\"content\":{\"blockPath\":[],\"channel\":[1,12],\"dimensions\":[12,12],\"domain\":\"\",\"leafPath\":\"MATLAB System1:2.eresult.P\",\"lineColor\":\"#4dbeee\",\"lineWidth\":2,\"parentID\":15,\"port\":1,\"sid\":[\"\"],\"signalID\":190,\"signalName\":\"MATLAB System1:2.eresult.P\"},\"type\":\"RecordBlkView.Signal\",\"uuid\":\"\"},{\"content\":{\"blockPath\":[],\"channel\":[2,12],\"dimensions\":[12,12],\"domain\":\"\",\"leafPath\":\"MATLAB System1:2.eresult.P\",\"lineColor\":\"#a2142f\",\"lineWidth\":2,\"parentID\":15,\"port\":1,\"sid\":[\"\"],\"signalID\":191,\"signalName\":\"MATLAB System1:2.eresult.P\"},\"type\":\"RecordBlkView.Signal\",\"uuid\":\"\"},{\"content\":{\"blockPath\":[],\"channel\":[3,12],\"dimensions\":[12,12],\"domain\":\"\",\"leafPath\":\"MATLAB System1:2.eresult.P\",\"lineColor\":\"#139fff\",\"lineWidth\":2,\"parentID\":15,\"port\":1,\"sid\":[\"\"],\"signalID\":192,\"signalName\":\"MATLAB System1:2.eresult.P\"},\"type\":\"RecordBlkView.Signal\",\"uuid\":\"\"},{\"content\":{\"blockPath\":[],\"channel\":[4,12],\"dimensions\":[12,12],\"domain\":\"\",\"leafPath\":\"MATLAB System1:2.eresult.P\",\"lineColor\":\"#ff6929\",\"lineWidth\":2,\"parentID\":15,\"port\":1,\"sid\":[\"\"],\"signalID\":193,\"signalName\":\"MATLAB System1:2.eresult.P\"},\"type\":\"RecordBlkView.Signal\",\"uuid\":\"\"},{\"content\":{\"blockPath\":[],\"channel\":[5,12],\"dimensions\":[12,12],\"domain\":\"\",\"leafPath\":\"MATLAB System1:2.eresult.P\",\"lineColor\":\"#b746ff\",\"lineWidth\":2,\"parentID\":15,\"port\":1,\"sid\":[\"\"],\"signalID\":194,\"signalName\":\"MATLAB System1:2.eresult.P\"},\"type\":\"RecordBlkView.Signal\",\"uuid\":\"\"},{\"content\":{\"blockPath\":[],\"channel\":[6,12],\"dimensions\":[12,12],\"domain\":\"\",\"leafPath\":\"MATLAB System1:2.eresult.P\",\"lineColor\":\"#64d413\",\"lineWidth\":2,\"parentID\":15,\"port\":1,\"sid\":[\"\"],\"signalID\":195,\"signalName\":\"MATLAB System1:2.eresult.P\"},\"type\":\"RecordBlkView.Signal\",\"uuid\":\"\"},{\"content\":{\"blockPath\":[],\"channel\":[7,12],\"dimensions\":[12,12],\"domain\":\"\",\"leafPath\":\"MATLAB System1:2.eresult.P\",\"lineColor\":\"#ff13a6\",\"lineWidth\":2,\"parentID\":15,\"port\":1,\"sid\":[\"\"],\"signalID\":196,\"signalName\":\"MATLAB System1:2.eresult.P\"},\"type\":\"RecordBlkView.Signal\",\"uuid\":\"\"},{\"content\":{\"blockPath\":[],\"channel\":[8,12],\"dimensions\":[12,12],\"domain\":\"\",\"leafPath\":\"MATLAB System1:2.eresult.P\",\"lineColor\":\"#fe330a\",\"lineWidth\":2,\"parentID\":15,\"port\":1,\"sid\":[\"\"],\"signalID\":197,\"signalName\":\"MATLAB System1:2.eresult.P\"},\"type\":\"RecordBlkView.Signal\",\"uuid\":\"\"},{\"content\":{\"blockPath\":[],\"channel\":[9,12],\"dimensions\":[12,12],\"domain\":\"\",\"leafPath\":\"MATLAB System1:2.eresult.P\",\"lineColor\":\"#22b573\",\"lineWidth\":2,\"parentID\":15,\"port\":1,\"sid\":[\"\"],\"signalID\":198,\"signalName\":\"MATLAB System1:2.eresult.P\"},\"type\":\"RecordBlkView.Signal\",\"uuid\":\"\"},{\"content\":{\"blockPath\":[],\"channel\":[10,12],\"dimensions\":[12,12],\"domain\":\"\",\"leafPath\":\"MATLAB System1:2.eresult.P\",\"lineColor\":\"#0072bd\",\"lineWidth\":2,\"parentID\":15,\"port\":1,\"sid\":[\"\"],\"signalID\":199,\"signalName\":\"MATLAB System1:2.eresult.P\"},\"type\":\"RecordBlkView.Signal\",\"uuid\":\"\"},{\"content\":{\"blockPath\":[],\"channel\":[11,12],\"dimensions\":[12,12],\"domain\":\"\",\"leafPath\":\"MATLAB System1:2.eresult.P\",\"lineColor\":\"#d95319\",\"lineWidth\":2,\"parentID\":15,\"port\":1,\"sid\":[\"\"],\"signalID\":200,\"signalName\":\"MATLAB System1:2.eresult.P\"},\"type\":\"RecordBlkView.Signal\",\"uuid\":\"\"},{\"content\":{\"blockPath\":[],\"channel\":[12,12],\"dimensions\":[12,12],\"domain\":\"\",\"leafPath\":\"MATLAB System1:2.eresult.P\",\"lineColor\":\"#edb120\",\"lineWidth\":2,\"parentID\":15,\"port\":1,\"sid\":[\"\"],\"signalID\":201,\"signalName\":\"MATLAB System1:2.eresult.P\"},\"type\":\"RecordBlkView.Signal\",\"uuid\":\"\"}]},\"type\":\"RecordBlkView.InputSignals\",\"uuid\":\"\"}],\"packageUris\":[\"http:\\/\\/schema.mathworks.com\\/mf0\\/streamout_blocks\\/R2020a\"],\"version\":\"1.0\"}"  VisualizationBindings="{\"sparklinesplugin\":{\"info\":[{\"bindingParametersList\":[],\"subplotID\":1}]}}"
  Scope : Scope  NumInputPorts=2
  Scope3 : Scope
  Unit Delay : UnitDelay  InitialCondition=x0  SampleTime=dt  HasFrameUpgradeWarning=on
  Zero-Order Hold : ZeroOrderHold  SampleTime=dt
  Scope1 : Scope
  wires:
  Plant/1 -> Scope3/1, Unit Delay/1  "state"
  Clock/1 -> Zero-Order Hold/1
  Zero-Order Hold/1 -> MATLAB System1/2
  MATLAB System1/1 -> Plant/1
  Unit Delay/1 -> MATLAB System1/1
  Bus Selector/1 -> Scope/1  "<p>"
  Bus Selector/2 -> Scope/2  "<state>"
  MATLAB System1/2 -> Record/1, Bus Selector/1
